simulink model "inverter_igbt_unipolar_spwm"  (R2024b)
settings: Solver=ode4  StartTime=0.0  StopTime=4/100  FixedStep=10e-6  RelTol=1e-3
libraries: spsMosfetLib x4, spsDCVoltageSourceLib x1, spsSeriesRLCBranchLib x1, spsTriangleGeneratorLib x1, spsVoltageMeasurementLib x1, sps_lib x1
settings Model: Creator=Abhijith_Kumble  LastModifiedBy=Abhijith_Kumble

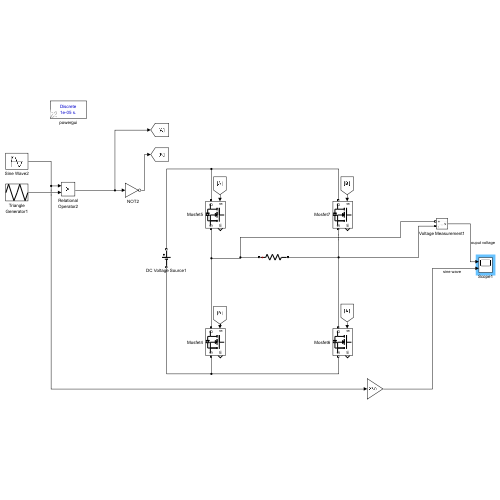
[thumbnail: Simulink's stored preview of the top-level diagram]
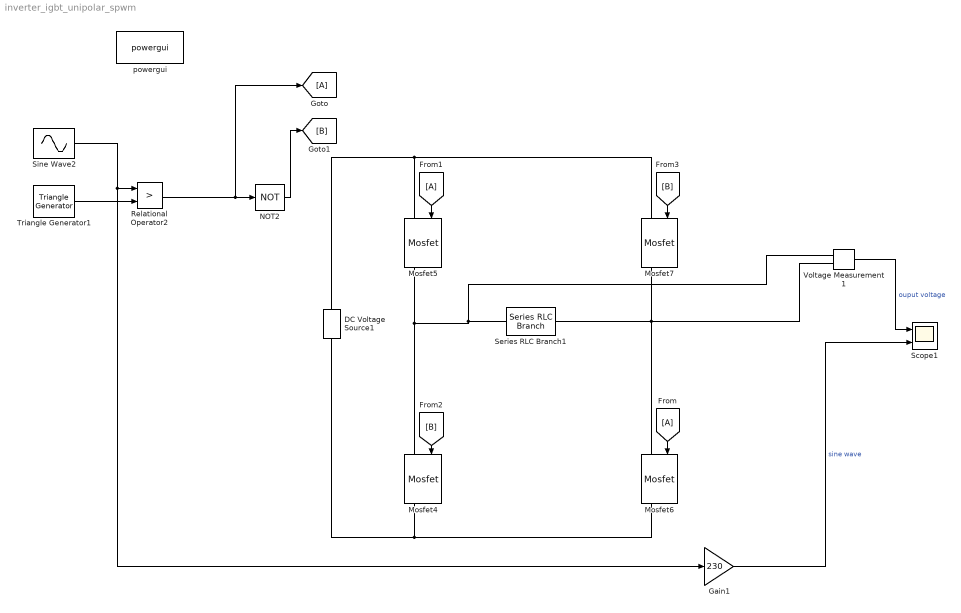
== system inverter_igbt_unipolar_spwm ==
  DC Voltage Source1 : spsDCVoltageSourceLib/DC Voltage Source  Amplitude=230  Measurements=None
  From : From
  From1 : From
  Gain1 : Gain  Gain=230
  Goto : Goto
  Mosfet{4..7} (4 alike) : spsMosfetLib/Mosfet  Ron=0.1  Lon=0  Rd=0.01  Vfd=0  IC=0  Rs=1e5  Cs=inf  Measurements=on
  NOT2 : Logic  Operator=NOT  IconShape=distinctive  AllPortsSameDT=off  OutDataTypeStr=boolean
  Relational Operator2 : RelationalOperator  Operator=>  OutDataTypeStr=boolean  RndMeth=Simplest  InputSameDT=off
  Scope1 : Scope  NumInputPorts=2
  Series RLC Branch1 : spsSeriesRLCBranchLib/Series RLC Branch  LConnTagsString=__new0  RConnTagsString=__new0  BranchType=R  Resistance=10  Inductance=1e-3  SetiL0=off  InitialCurrent=0  Capacitance=1e-6  Setx0=off  InitialVoltage=0  Measurements=None
  Sine Wave2 : Sin  Frequency=2*pi*50  SampleTime=0
  Triangle Generator1 : spsTriangleGeneratorLib/Triangle Generator  Freq=1e3  Phase=90  Ts=0
  Voltage Measurement1 : spsVoltageMeasurementLib/Voltage Measurement  PhasorSimulation=off  OutputType=Complex  PSBequivalent=0
  powergui : sps_lib/powergui  Priority=1  SimulationMode=Discrete  SampleTime=10e-6  frequency=60  Iterations=50  frequencyindice=0  Pbase=100e6  ErrMax=1e-4  UnitsV=kV  UnitsW=MW  buscounter=0  FunctionMessages=off  echomessages=off  EnableUseOfTLC=off  CurrentSourceSwitches=off  DisableSnubberDevices=off  DisableRonSwitches=off  DisableVfSwitches=off  DisplayEquations=off  AutomaticDiscreteSolvers=off  SolverType=Tustin/Backward Euler (TBE)  Interpol=off  ExternalGateDelay=off  methode=off  Ts=100  x0status=blocks  SPID=on  SwTol=0  HookPort=off  NonlinearTolerance=1e-4  nMaxIteration=100  ContinueOnMaxIteration=off  RestoreLinks=warning  ResistiveCurrentMeasurement=off  Frange=[0:2:500]  Ylog=off  Xlog=on  ShowGrid=off  save=off  variable=ZData  structure=0  ZoomFFT=off  StartTime=0.0  cycles=1  DisplayStyle=1  fundamental=60  FreqAxis=off  MaxFrequency=1000  frequencyindicesteady=1  RmsSteady=1  display=off
  wires:
  Voltage Measurement1/1 -> Scope1/1  "ouput voltage"
  Sine Wave2/1 -> Gain1/1, Relational Operator2/1
  NOT2/1 -> [B]
  [B] -> Mosfet4/1
  From/1 -> Mosfet6/1
  From1/1 -> Mosfet5/1
  Triangle Generator1/1 -> Relational Operator2/2
  [B] -> Mosfet7/1
  Relational Operator2/1 -> Goto/1, NOT2/1
  Gain1/1 -> Scope1/2  "sine wave"
  connections:
  Mosfet7/LConn1 -- DC Voltage Source1/RConn1 -- Mosfet5/LConn1
  Series RLC Branch1/RConn1 -- Voltage Measurement1/LConn2 -- Mosfet7/RConn1 -- Mosfet6/LConn1
  Series RLC Branch1/LConn1 -- Voltage Measurement1/LConn1 -- Mosfet4/LConn1 -- Mosfet5/RConn1
  DC Voltage Source1/LConn1 -- Mosfet6/RConn1 -- Mosfet4/RConn1
